simulink model "parallele_ECS_Stock_aval"  (R2024b)
settings: Solver=FixedStepAuto  StartTime=0.0  StopTime=1436400  FixedStep=300  RelTol=1e-3
settings Model: Creator=mouzounb  LastModifiedBy=mouzounb
settings DataIOCC: ExternalInput=feuille.getElement('m_ch_dir'),feuille.getElement('m_ECS_sout'),feuille.getElement('m_ECS_stock'),feuille.getElement('m_ECS_sec'),feuille.getElement('m_ch_V3V'),feuille.getElement('m_prim'),feuille.getElement('T_prim_in'),feuille.getElement('T_edv'),feuille.getElement('m_ECS_dir'),feuille.getElement('m_ECS_V3V'),feuille.getElement('m_ECS_bouc')  LoadExternalInput=on
settings OptimizationCC: StrengthReduction=on  PassReuseOutputArgsAs=Individual arguments  OptimizeBlockOrder=speed  OptimizationPriority=Speed  OptimizationCustomize=off  MultiThreadedLoops=on  AutoScheduleForLoops=on  EfficientTunableParamExpr=on
settings DebuggingCC: ParameterTunabilityLossMsg=error
settings RTWCC: Description=Embedded Coder  SystemTargetFile=ert.tlc  TemplateMakefile=ert_default_tmf  BuildConfiguration=Faster Runs  CodeProfilingInstrumentation=coarse
settings CodeAppCC: ForceParamTrailComments=on  IgnoreCustomStorageClasses=off  OperatorAnnotations=on  SimulinkDataObjDesc=on  SFDataObjDesc=on  ParamNamingRule=UpperCase  InsertBlockDesc=on  BlockCommentType=BlockSIDComment  MATLABSourceComments=on
settings ERTTargetCC: TargetLangStandard=C99 (ISO)  GenerateSampleERTMain=on  SupportComplex=off  SupportContinuousTime=on  SupportVariableSizeSignals=on  InlinedParameterPlacement=Hierarchical  ERTCustomFileTemplate=example_file_process.tlc  RateTransitionBlockCode=Function  IndentStyle=Allman

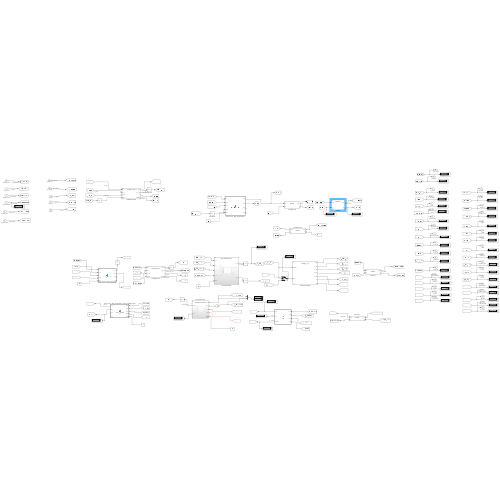
[thumbnail: Simulink's stored preview of the top-level diagram]
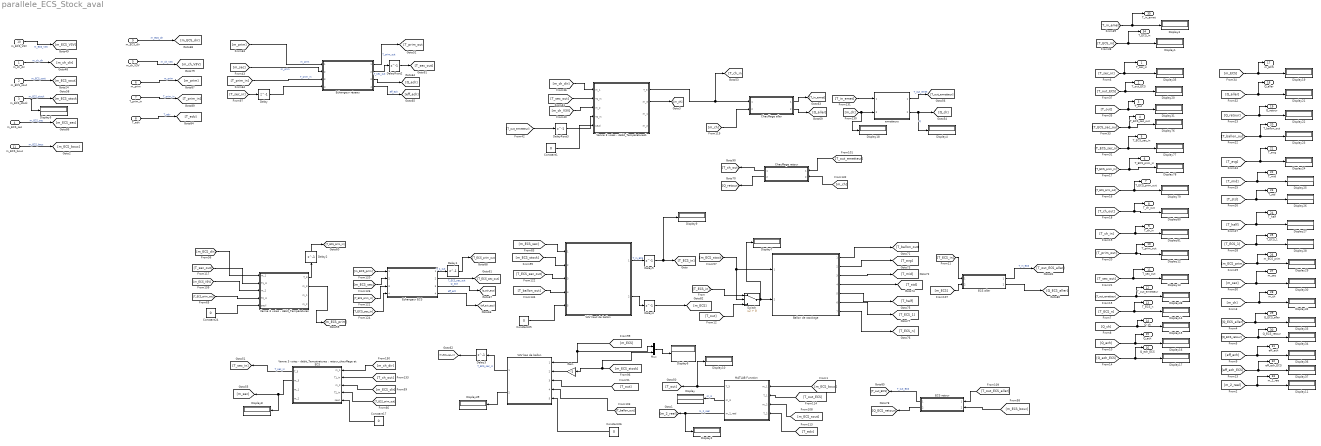
== system parallele_ECS_Stock_aval ==
  m_ch_dir : Inport
  m_ECS_sout : Inport  Port=2
  m_ECS_stock : Inport  Port=3  Interpolate=off
  m_ECS_sec : Inport  Port=4
  m_ch_V3V : Inport  Port=5
  m_prim : Inport  Port=6
  T_prim_in : Inport  Port=7
  T_edv : Inport  Port=8
  m_ECS_dir : Inport  Port=9
  m_ECS_V3V : Inport  Port=10
  m_ECS_bouc : Inport  Port=11
  Ballon de stockage : Subsystem  ReferencedSubsystem=stockage_T_C  D=1  H=1.5  n=61  V_var=60  V_min=10  U=5  eps=2  T_amb=20
  Chauffage aller : Subsystem  ReferencedSubsystem=conduite  m_min=0.1  classe_iso=4  D=0.15  L=50  T_local=15
  Chauffage retour : Subsystem  ReferencedSubsystem=conduite  m_min=0.1  classe_iso=4  D=0.15  L=50  T_local=15
  Constant{1,17,24..26} (5 alike) : Constant  Value=0
  Delay{,1..5} (6 alike) : Delay  DelayLength=1  InputProcessing=Columns as channels (frame based)
  DelayRoot2 : Delay  DelayLength=1  InputProcessing=Columns as channels (frame based)
  DelayRoot3 : Delay  DelayLength=1  InputProcessing=Columns as channels (frame based)
  Display{,1..39,76..81} (46 alike) : Display
  ECS aller : Subsystem  ReferencedSubsystem=conduite  m_min=0.1  classe_iso=4  D=0.03  L=50  T_local=15
  ECS retour : Subsystem  ReferencedSubsystem=conduite  m_min=0.1  classe_iso=4  D=0.03  L=50  T_local=15
  Echangeur ECS : Subsystem  ReferencedSubsystem=echangeur_NUT  U=1000  S=100
  Echangeur réseau : Subsystem  ReferencedSubsystem=echangeur_NUT  U=1000  S=100
  Gain : Gain  Gain=-1
  MATLAB Function : MATLAB Function  TreatAsAtomicUnit=on
  Mux : Mux  Inputs=2
  Switch : Switch  Criteria=u2 > Threshold  SaturateOnIntegerOverflow=off  InputSameDT=off
  V3V bas de ballon : Subsystem  ReferencedSubsystem=V3V_bifonctions_ECS
  V3V haut de ballon : Subsystem  ReferencedSubsystem=V3V_bifonctions_ECS
  Vanne 3 voies - débit_Températures : MATLAB Function  TreatAsAtomicUnit=on
  "Vanne 3 voies - débit_Températures : retour_chauffage et ECS" : MATLAB Function  TreatAsAtomicUnit=on
  Vanne 3 voies - débit_Températures1 : MATLAB Function  TreatAsAtomicUnit=on
  emetteurs : Subsystem  ReferencedSubsystem=emetteurs  m_min=0.1  n_radiateurs=12  n_tubes=2  D=0.02  L=3  U=50  T_air=20
  T_sec_in : Outport
  T_out_ECS : Outport  Port=2
  T_out : Outport  Port=3
  T_ECS_sec_out : Outport  Port=4
  T_ECS_sec_in : Outport  Port=5
  T_ECS_prim_in : Outport  Port=6
  T_ECS_prim_out : Outport  Port=7
  T_ch_out : Outport  Port=8
  T_ch_in : Outport  Port=9
  T_prim_out : Outport  Port=10
  T_sec_out : Outport  Port=11
  T_out_emetteur : Outport  Port=12
  T_ECS_n : Outport  Port=13
  Q_ch : Outport  Port=14
  Q_ech : Outport  Port=15
  Q_ech_ECS : Outport  Port=16
  m_ECS : Outport  Port=17
  Q_aller : Outport  Port=18
  Q_retour : Outport  Port=19
  T_ballon_out : Outport  Port=20
  T_avg : Outport  Port=21
  T_mid : Outport  Port=22
  T_std : Outport  Port=23
  T_half : Outport  Port=24
  T_ECS_1 : Outport  Port=25
  m_ECS_prim : Outport  Port=26
  m_sec : Outport  Port=27
  m_ch : Outport  Port=28
  Q_ECS_aller : Outport  Port=29
  Q_ECS_retour : Outport  Port=30
  eff_ech : Outport  Port=31
  eff_ech_ECS : Outport  Port=32
  m_2_ree : Outport  Port=33
  T_ECS_in : Outport  Port=34
  T_in_emet : Outport  Port=35
  wires:
  Gain/1 -> V3V bas de ballon/2
  V3V bas de ballon/1 -> Delay3/1  "T_ECS_sec_in"
  [T_ballon_out] -> V3V bas de ballon/4
  V3V bas de ballon/2 -> Display39/1
  Constant25/1 -> V3V haut de ballon/5
  V3V haut de ballon/1 -> Delay5/1  "T_in_ECS"
  [T_ballon_out] -> V3V haut de ballon/4
  [m_ECS_stock] -> V3V haut de ballon/2
  [m_ECS_sec] -> V3V haut de ballon/1
  Mux/1 -> Display6/1
  Constant26/1 -> V3V bas de ballon/5
  [T_ECS_prim_out] -> Vanne 3 voies - débit_Températures/4(T2_in)
  Ballon de stockage/4 -> [T_std]
  [T_prim_in] -> Echangeur réseau/3  "T_prim_in"
  Constant24/1 -> Vanne 3 voies - débit_Températures/5(seuil)
  emetteurs/1 -> [T_out_emetteur]  "T_out_emet"
  Ballon de stockage/5 -> [T_half]
  ECS aller/1 -> [T_out_ECS_aller]  "T_in_ECS"
  [m_ECS] -> ECS aller/2
  Echangeur ECS/4 -> [eff_ech_ECS]  "eff_ech"
  Ballon de stockage/6 -> [T_ECS_1]
  Echangeur réseau/3 -> [Q_ech]
  [m_prim] -> Echangeur réseau/1  "m_prim"
  [m_ECS_prim] -> Echangeur ECS/1
  [m_ECS_stock] -> Gain/1, Mux/2
  Ballon de stockage/2 -> [T_avg]
  [T_ECS_in] -> ECS aller/1
  [m_ECS_dir] -> Vanne 3 voies - débit_Températures/1("m_1 ")
  [T_sec_out] -> Vanne 3 voies - débit_Températures/2(T1_in)
  Ballon de stockage/3 -> [T_mid]
  [m_ECS_sout] -> MATLAB Function/3(m_2)
  Vanne 3 voies - débit_Températures/2(m_3) -> [m_ECS_prim]
  Echangeur ECS/3 -> [Q_ech_ECS]  "Q_ech"
  Constant17/1 -> "Vanne 3 voies - débit_Températures : retour_chauffage et ECS"/5(seuil)
  [m_ECS_sec] -> Echangeur ECS/2
  Delay/1 -> Echangeur réseau/4
  [T_out] -> V3V bas de ballon/3
  Echangeur réseau/2 -> DelayRoot2/1  "T_sec_out"
  [m_ch_dir] -> "Vanne 3 voies - débit_Températures : retour_chauffage et ECS"/1("m_1 ")
  MATLAB Function/3(m_2_reel) -> Display2/1, [m_2_reel]  "m_2_reel"
  [m_ch] -> emetteurs/2, Display18/1
  Echangeur ECS/1 -> Delay1/1  "T_1_out"
  [T_edv] -> MATLAB Function/4(T_2)
  emetteurs/2 -> Display4/1, [Q_ch]  "Q"
  [T_out_ECS] -> MATLAB Function/2(T_1)
  [T_ch_out] -> "Vanne 3 voies - débit_Températures : retour_chauffage et ECS"/2(T1_in)
  [T_ECS_prim_in] -> Echangeur ECS/3
  "Vanne 3 voies - débit_Températures : retour_chauffage et ECS"/1(T_3) -> [T_sec_in]  "T_sec_in"
  ECS retour/1 -> [T_out_ECS]  "T_out_ECS"
  [T_ECS_prim_out] -> "Vanne 3 voies - débit_Températures : retour_chauffage et ECS"/4(T2_in)
  MATLAB Function/2(m_3) -> Display/1  "m_3"
  [T_sec_in] -> Delay/1
  Vanne 3 voies - débit_Températures/1(T_3) -> Delay2/1
  Echangeur réseau/4 -> [eff_ech]  "eff_ech"
  [T_out_ECS_aller] -> ECS retour/1
  MATLAB Function/1(T_3) -> Display10/1, [T_out]
  Echangeur ECS/2 -> [T_ECS_sec_out]  "T_ECS_sec_out"
  [m_ECS_V3V] -> Vanne 3 voies - débit_Températures/3("m_2 ")
  [m_ECS] -> V3V bas de ballon/1, Mux/1
  Ballon de stockage/1 -> [T_ballon_out]
  [m_ECS_bouc] -> ECS retour/2
  Ballon de stockage/7 -> [T_ECS_n]
  [T_ECS_sec_in] -> Echangeur ECS/4
  Echangeur réseau/1 -> [T_prim_out]  "T_prim_out"
  [T_in_emet] -> emetteurs/1
  [m_ECS_dir] -> "Vanne 3 voies - débit_Températures : retour_chauffage et ECS"/3("m_2 ")
  [T_ECS_sec_out] -> V3V haut de ballon/3
  "Vanne 3 voies - débit_Températures : retour_chauffage et ECS"/2(m_3) -> Display8/1, [m_sec]
  DelayRoot2/1 -> [T_sec_out]
  Delay1/1 -> [T_ECS_prim_out]
  Delay2/1 -> [T_ECS_prim_in]
  Delay3/1 -> [T_ECS_sec_in]
  [T_out] -> Switch/3
  [m_ECS_stock] -> Ballon de stockage/1, Switch/2
  Switch/1 -> Display7/1, Ballon de stockage/2
  m_prim/1 -> [m_prim]  "m_prim"
  m_ECS_stock/1 -> Display5/1, [m_ECS_stock]  "m_ECS_stock"
  T_prim_in/1 -> [T_prim_in]  "T_prim_in"
  m_ECS_dir/1 -> [m_ECS_dir]  "m_ECS_dir"
  T_edv/1 -> [T_edv]  "T_edv"
  m_ECS_sout/1 -> [m_ECS_sout]  "m_ECS_sout"
  m_ECS_sec/1 -> [m_ECS_sec]  "m_ECS_sec"
  m_ECS_V3V/1 -> [m_ECS_V3V]  "m_ECS_V3V"
  m_ch_V3V/1 -> [m_ch_V3V]  "m_ch_V3V"
  m_ch_dir/1 -> [m_ch_dir]  "m_ch_dir"
  [T_ch_in] -> T_ch_in/1, Display81/1
  [T_std] -> T_std/1, Display26/1
  [Q_ECS_retour] -> Q_ECS_retour/1, Display34/1
  [Q_aller] -> Q_aller/1, Display21/1
  [T_ECS_n] -> T_ECS_n/1, Display14/1
  [eff_ech_ECS] -> eff_ech_ECS/1, Display37/1
  [T_half] -> T_half/1, Display27/1
  [T_sec_in] -> Display35/1, T_sec_in/1
  [m_ECS] -> m_ECS/1, Display19/1
  [m_2_reel] -> m_2_ree/1, Display11/1
  [T_out_ECS] -> T_out_ECS/1, Display20/1
  [Q_ECS_aller] -> Q_ECS_aller/1, Display33/1
  [T_out] -> T_out/1, Display31/1
  [T_mid] -> T_mid/1, Display25/1
  [m_sec] -> m_sec/1, Display30/1
  [Q_ech] -> Q_ech/1, Display16/1
  [eff_ech] -> eff_ech/1, Display36/1
  [T_avg] -> T_avg/1, Display24/1
  [T_ECS_sec_in] -> T_ECS_sec_in/1, Display77/1
  [T_sec_out] -> T_sec_out/1, Display13/1
  [T_ch_out] -> T_ch_out/1, Display80/1
  [T_ECS_prim_in] -> T_ECS_prim_in/1, Display78/1
  [m_ch] -> m_ch/1, Display32/1
  [T_prim_out] -> T_prim_out/1, Display12/1
  [Q_ch] -> Q_ch/1, Display15/1
  [Q_retour] -> Q_retour/1, Display22/1
  [T_ECS_1] -> T_ECS_1/1, Display28/1
  [T_ECS_sec_out] -> T_ECS_sec_out/1, Display76/1
  [Q_ech_ECS] -> Q_ech_ECS/1, Display17/1
  [T_out_emetteur] -> T_out_emetteur/1, Display38/1
  [T_ballon_out] -> T_ballon_out/1, Display23/1
  [T_ECS_prim_out] -> T_ECS_prim_out/1, Display79/1
  [m_ECS_prim] -> m_ECS_prim/1, Display29/1
  [m_ECS_bouc] -> MATLAB Function/1(m_1)
  ECS retour/2 -> [Q_ECS_retour]
  ECS aller/2 -> [Q_ECS_aller]
  V3V haut de ballon/2 -> Delay4/1
  Delay4/1 -> [m_ECS]
  Vanne 3 voies - débit_Températures1/1(T_3) -> [T_ch_in], Chauffage aller/1
  Chauffage aller/1 -> [T_in_emet]
  [T_out_emetteur] -> Chauffage retour/1
  [m_ch] -> Chauffage retour/2
  Chauffage retour/1 -> [T_ch_out]
  [m_ch] -> Chauffage aller/2
  [T_ECS_in] -> Switch/1
  Delay5/1 -> Display9/1, [T_ECS_in]
  [T_ECS_in] -> T_ECS_in/1, Display1/1
  [T_in_emet] -> Display3/1, T_in_emet/1
  Chauffage retour/2 -> [Q_retour]
  Chauffage aller/2 -> [Q_aller]
  m_ECS_bouc/1 -> [m_ECS_bouc]  "m_ECS_bouc"
  [m_ch_dir] -> Vanne 3 voies - débit_Températures1/1("m_1 ")
  [m_ch_V3V] -> Vanne 3 voies - débit_Températures1/3("m_2 ")
  [T_sec_out] -> Vanne 3 voies - débit_Températures1/2(T1_in)
  [T_out_emetteur] -> DelayRoot3/1
  Vanne 3 voies - débit_Températures1/2(m_3) -> [m_ch]
  Constant1/1 -> Vanne 3 voies - débit_Températures1/5(seuil)
  [m_sec] -> Echangeur réseau/2  "m_prim"
  DelayRoot3/1 -> Vanne 3 voies - débit_Températures1/4(T2_in)

== matlab function parallele_ECS_Stock_aval/MATLAB Function ==
  data: m_1 input size=1; T_3 output size=1; T_1 input size=1; m_2 input size=1; T_2 input size=1; m_3 output size=1; m_2_reel output size=1
function [T_3, m_3, m_2_reel] = fcn(m_1, T_1, m_2, T_2)
% DESCRIPTION
% Vanne 3 voies de mélange. Rassemble les flux suivants:
% - retour bouclage ECS: débit m_1 [kg/s] à la température T_1 [°C]
% - eau froide du réseau de la ville pour compenser les soutirages: débit m_2 [kg/s] (débit de soutirage consigne)
%    - Si le débit d'aller ECS est suffisant (m1>=0), ce débit m_2 est aussi le débit
%   de soutirage réel (m_2_reel).
%   La consigne de soutirage est respectée: consigne = réel.
%    - Sinon (m_1<0), il est corrigé pour correspondre à l'eau qui a été vraiment soutirée.
%   Ce nouveau m_2_reel (soutirage réel) est comparé au m_2 soutirage consigne
%   au niveau pilotage pour pénalisation.
% 
% REMARQUE
% si m_1 > 0 mais m_1 est trop faible, la température T_1 ne
% respecte pas la consigne légionelles (par exemple T_1 > 53°C). Ceci:
%   - ne change pas le comportement de la vanne
%   - est pénalisé au niveau pilotage en comparant T_1 à la consigne.
%
% SORTIES
% - Le flux 3 de débit m_3 [kg/s] à la température T_3 [°C], qui est un
% mélange des flux 1 et 2. m_3 est aussi le débit d'ECS aller.
% - Le débit de soutirage réel m_2 [kg/s], qui peut etre égal ou inférieur ou débit de
% soutirage consigne
%
% HYPOTHESES
% - Les capacités calorifiques des fluides 1 et 2 sont identiques (Cp_1 =
% Cp_2)
% - Si m_3 est presque nul (ou nul), on retient la moyenne des températures pour T_3.


    if m_1 < 0
        % si le débit aller du bouclage est trop faible, le soutirage ne peut
        % etre réalisé complètement:
        % - il revient un débit m_1 négatif 
        % qui révèle que seulement m_2 - abs(m_1) a été réellement soutiré
        % - donc le débit soutirage m_2 consigne est actualisé en m_2_reel, c'est le meme débit qui
        % est utilisé pour l'arrivé d'eau froide
        % 
        % remarque: m_2 - abs(m_1) ne peut etre négatif car le débit aller du
        % bouclage est positif et m_2 (soutirage consigne) est imposé positif
        m_2_reel = m_2 - abs(m_1);
    else
        m_2_reel = m_2;
    end
    
    m_1 = max(m_1, 0);    
    m_3 = m_1 + m_2_reel;
    if m_3 == 0
        T_3 = (T_1 + T_2) / 2;
    else
        T_3 = (m_1 * T_1 + m_2_reel * T_2) / m_3;
    end

end

== matlab function parallele_ECS_Stock_aval/Vanne 3 voies - débit_Températures1 ==
  data: m_1 input; T1_in input; m_2 input; T_3 output; T2_in input; m_3 output; m_1 output; m_2 output; seuil input
% Fonction de la vanne 3 voies 
function [T_3, m_3,m_1, m_2 ] = vanne_3_voies(m_1, T1_in, m_2, T2_in, seuil)
    % Vérification que le débit total n'est pas nul
    m_1 = max(0, m_1);
    m_2 = max(0, m_2);
m_3 = m_1 + m_2;
if m_3 < seuil
    m_1 = 0;
    m_2 = 0;
    m_3 = 0;
end
Cp_1 = 4180; % J/(kg.K)
Cp_2 = 4180; % J/(kg.K)

if m_2 == 0 && m_1 == 0
    m_1 = 1;
    m_2 = 1;
end
F_1 = m_1 * Cp_1;
F_2 = m_2 * Cp_2;
   % Calcul de la température du mélange
T_3 = (T1_in* F_1 + T2_in * F_2 )/(F_1 + F_2);

end
% Calcul de la température du mélange en sortie
% T_out = (mdot1 * T1_in + mdot2 * T2_in) / mdot_out;

== matlab function parallele_ECS_Stock_aval/Vanne 3 voies - débit_Températures : retour_chauffage et ECS ==
  data: m_1 input; T1_in input; m_2 input; T_3 output; T2_in input; m_3 output; m_1 output; m_2 output; seuil input
% Fonction de la vanne 3 voies 
function [T_3, m_3,m_1, m_2 ] = vanne_3_voies(m_1, T1_in, m_2, T2_in, seuil)
    % Vérification que le débit total n'est pas nul
    m_1 = max(0, m_1);
    m_2 = max(0, m_2);
m_3 = m_1 + m_2;
if m_3 < seuil
    m_1 = 0;
    m_2 = 0;
    m_3 = 0;
end
Cp_1 = 4180; % J/(kg.K)
Cp_2 = 4180; % J/(kg.K)

m_1 = max(m_1, 0);
m_2 = max(m_2, 0);

if m_2 == 0 && m_1 == 0
    m_1 = 1;
    m_2 = 1;
end
F_1 = m_1 * Cp_1;
F_2 = m_2 * Cp_2;
   % Calcul de la température du mélange
T_3 = (T1_in * F_1 + T2_in * F_2 )/(F_1 + F_2);

end
% Calcul de la température du mélange en sortie
% T_out = (mdot1 * T1_in + mdot2 * T2_in) / mdot_out;

== matlab function parallele_ECS_Stock_aval/Vanne 3 voies - débit_Températures ==
  data: m_1 input; T1_in input; m_2 input; T_3 output; T2_in input; m_3 output; m_1 output; m_2 output; seuil input
% Fonction de la vanne 3 voies 
function [T_3, m_3,m_1, m_2 ] = vanne_3_voies(m_1, T1_in, m_2, T2_in, seuil)
    % Vérification que le débit total n'est pas nul
    m_1 = max(0, m_1);
    m_2 = max(0, m_2);
m_3 = m_1 + m_2;
if m_3 < seuil
    m_1 = 0;
    m_2 = 0;
    m_3 = 0;
end
Cp_1 = 4180; % J/(kg.K)
Cp_2 = 4180; % J/(kg.K)

if m_2 == 0 && m_1 == 0
    m_1 = 1;
    m_2 = 1;
end
F_1 = m_1 * Cp_1;
F_2 = m_2 * Cp_2;
   % Calcul de la température du mélange
T_3 = (T1_in* F_1 + T2_in * F_2 )/(F_1 + F_2);

end
% Calcul de la température du mélange en sortie
% T_out = (mdot1 * T1_in + mdot2 * T2_in) / mdot_out;
